simulink model "simulation_test"  (R2024a)
settings: Solver=VariableStepAuto  StartTime=0.0  StopTime=100  RelTol=1e-3
settings Model: Creator=mccat  LastModifiedBy=mccat

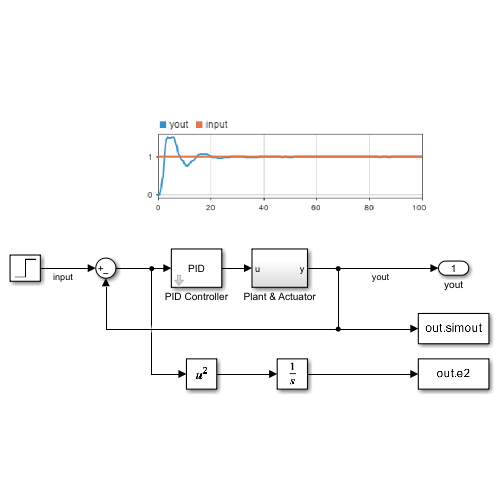
[thumbnail: Simulink's stored preview of the top-level diagram]
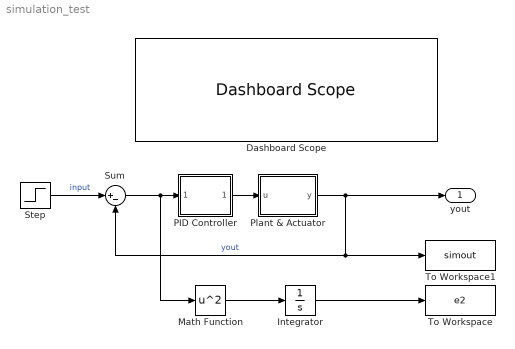
== system simulation_test ==
  Dashboard Scope : DashboardScope
  Integrator : Integrator
  Math Function : Math  Operator=square  SignedPower=on
  PID Controller : Subsystem  mask(PID Controller){P=0.91066, I=0.57075, D=1.427}
      mask prompts: P "Proportional:"; I "Integral"; D "Derivative:"
      mask help: Enter expressions for proportional, integral, and derivative terms.
      mask Help: This block implements a PID controller where paramaters are entered for the Proportional, Integral and Derivative terms.
      mask Display: disp('PID')
  Plant & Actuator : Subsystem
  Step : Step  Time=0  SampleTime=0
  Sum : Sum  Inputs=|+-  InputSameDT=on  SaturateOnIntegerOverflow=on  OutDataTypeStr=Inherit: Same as first input
  To Workspace : ToWorkspace  VariableName=e2  SampleTime=-1
      settings: MaxDataPoints=1
  To Workspace1 : ToWorkspace  VariableName=simout  SaveFormat=Structure With Time  SampleTime=-1
      settings: MaxDataPoints=1
  yout : Outport
  wires:
  Sum/1 -> PID Controller/1(input), Math Function/1
  Plant & Actuator/1(y) -> yout/1, To Workspace1/1, Sum/2  "yout"
  Integrator/1 -> To Workspace/1
  Math Function/1 -> Integrator/1
  PID Controller/1(output) -> Plant & Actuator/1("u ")
  Step/1 -> Sum/1  "input"

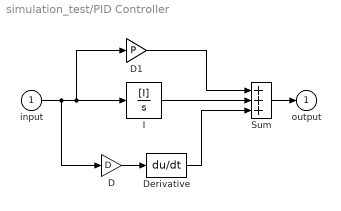
== system simulation_test/PID Controller ==
  input : Inport
  D : Gain  Gain=D  SaturateOnIntegerOverflow=on  OutDataTypeStr=Inherit: Same as input  ParamDataTypeStr=Inherit: Same as input
  D1 : Gain  Gain=P  SaturateOnIntegerOverflow=on  OutDataTypeStr=Inherit: Same as input  ParamDataTypeStr=Inherit: Same as input
  Derivative : Derivative
  I : TransferFcn  Numerator=[I]  Denominator=[1 0]
  Sum : Sum  Inputs=+++  InputSameDT=on  SaturateOnIntegerOverflow=on  OutDataTypeStr=Inherit: Same as first input
  output : Outport  InitialOutput=0
  wires:
  input/1 -> D1/1, I/1, D/1
  Sum/1 -> output/1
  D/1 -> Derivative/1
  Derivative/1 -> Sum/3
  I/1 -> Sum/2
  D1/1 -> Sum/1

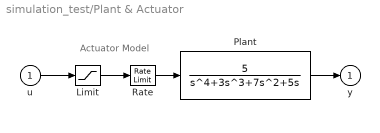
== system simulation_test/Plant & Actuator ==
  note: Actuator Model
  "u " : Inport
  Limit : Saturate  UpperLimit=2  LowerLimit=-2
  Plant : TransferFcn  Numerator=[5]  Denominator=[1 3 7 5 0]
  Rate : RateLimiter  RisingSlewLimit=0.8  FallingSlewLimit=-0.8
  y : Outport  InitialOutput=0
  wires:
  Plant/1 -> y/1
  "u "/1 -> Limit/1
  Rate/1 -> Plant/1
  Limit/1 -> Rate/1
